simulink model "ultra"  (R2020b)
settings: Solver=FixedStepDiscrete  StartTime=0.0  StopTime=10.0  FixedStep=0.0005  RelTol=1e-3  EnableMultiTasking=on
undefined symbols (not defined in the file): acc_calmax1, acc_calmax2, acc_calmin1, acc_calmin2, akemancanshu, bre, bre_calmax, bre_calmin, ecucoder_acal, I_AN01_5K1, I_AN03_5V, I_AN04_5V, kd, ki, kp, leftmax, O_SW06_HS1A, rightmax, T_add, T_del, tiaoshi, zhiling
libraries: ec5744lib x215, canmsglib x75, simulink x10
(part 2 of 7)

== system ultra/RX/转向——receive编码器 ==
  CANReceive1 : ec5744lib/RapidECU_U4B/04CANCommunication/CANReceive  canmodule=1  canbuffer=55  canmessageid=hex2dec('99')  canmessagetype=Standard(11-bit ID)  datalength=8  sampletime=-1
      settings: SourceProductName=ECUCoder for MPC5744
  MeaModule8 : ec5744lib/RapidECU_U4B/07Calibration/MeaModule  signal=CANOK_99
      settings: SourceProductName=ECUCoder for MPC5744
  Subsystem3 : Subsystem
  Terminator3 : Terminator
  wires:
  CANReceive1/1 -> Subsystem3/Trigger
  CANReceive1/4 -> Subsystem3/3(msg)
  CANReceive1/2 -> MeaModule8/1
  CANReceive1/5 -> Terminator3/1
  MeaModule8/1 -> Subsystem3/1(Enable)
  CANReceive1/3 -> Subsystem3/2(ID)

== system ultra/TOWORKSTATION/toworkstation ==
  Enable : EnablePort
  toworkstation : Subsystem

== system ultra/TOWORKSTATION/转向 ==
  Data Store Read : DataStoreRead  DataStoreName=match_model
  MATLAB Function : MATLAB Function  TreatAsAtomicUnit=on
  Subsystem : Subsystem
  wires:
  Data Store Read/1 -> MATLAB Function/1(u)
  MATLAB Function/1(y) -> Subsystem/Enable

== system ultra/TX控制器/Subsystem ==
  Enable : EnablePort
  CAN Pack1 : canmsglib/CAN Pack  Commented=on  CANdbFile=C:\Users\Liu keliang\Desktop\HRT2023\HRT23赛季刘科良\CANdbc\steere.dbc  MsgList=New_Message_1  MsgName=New_Message_1  MsgIDType=Standard (11-bit identifier)  MsgIdentifier=1911  MsgLength=4  Remote=off  ApplyMinMax=off  BusOutput=off  SignalInfo={'huahaizhuanxiangerror','16','16','LE','signed','Standard','0','1','0','-Inf','Inf';'steere','0','16','LE','signed','Standard','0','1','0','-Inf','Inf'}
      settings: SourceProductBaseCode=ME,XP,VN  DataFormat=CANdb specified signals
  CANPackMessage1 : ec5744lib/RapidECU_U4B/04CANCommunication/CANPackMessage  Commented=on  datalength=4  sampletime=-1
      settings: SourceProductName=ECUCoder for MPC5744
  CANTransmit1 : ec5744lib/RapidECU_U4B/04CANCommunication/CANTransmit  Commented=on  canmodule=2  canbuffer=15  canmessageid=hex2dec('777')  canmessagetype=Standard(11-bit ID)  datalength=4  sampletime=-1
      settings: SourceProductName=ECUCoder for MPC5744
  Data Store Read : DataStoreRead  Commented=on  DataStoreName=huahaisteere
  Data Store Read3 : DataStoreRead  Commented=on  DataStoreName=steere
  Data Type Conversion1 : DataTypeConversion  Commented=on  OutDataTypeStr=uint8
  Terminator1 : Terminator  Commented=on
  wires:
  Data Type Conversion1/1 -> CANTransmit1/1
  CANPackMessage1/1 -> Data Type Conversion1/1
  Data Store Read3/1 -> CAN Pack1/1
  CAN Pack1/1 -> CANPackMessage1/1
  CANTransmit1/1 -> Terminator1/1
  Data Store Read/1 -> CAN Pack1/2

== system ultra/TX控制器/Subsystem1 ==
  angle : Inport
  v : Inport  Port=2
  Data Store Read4 : DataStoreRead  DataStoreName=match_model
  ECCalVar : Constant  InitFcn=ecucoder_acal;  Value=akemancanshu  OutDataTypeStr=Inherit: Inherit via back propagation  SampleTime=-1
  MATLAB Function2 : MATLAB Function  TreatAsAtomicUnit=on
  youqianvvv : Outport
  zuoqianvvv : Outport  Port=2
  youhouvvv : Outport  Port=3
  zuohouvvv : Outport  Port=4
  wires:
  MATLAB Function2/2(zuoqianvvv) -> zuoqianvvv/1
  v/1 -> MATLAB Function2/2(v)
  MATLAB Function2/1(youqianvvv) -> youqianvvv/1
  MATLAB Function2/3(youhouvvv) -> youhouvvv/1
  angle/1 -> MATLAB Function2/1(anglenb)
  MATLAB Function2/4(zuohouvvv) -> zuohouvvv/1
  Data Store Read4/1 -> MATLAB Function2/3(model)
  ECCalVar/1 -> MATLAB Function2/4(k)

== system ultra/TX控制器/扭矩 ==
  Enable : EnablePort
  184左前 : Subsystem
  185右前 : Subsystem
  188右后 : Subsystem
  189左后 : Subsystem
  TEST : Subsystem

== system ultra/TX控制器/速度 ==
  Enable : EnablePort
  184左前 : Subsystem
  185右前 : Subsystem
  188右后 : Subsystem
  189左后 : Subsystem

== system ultra/esc,ABS/Subsystem ==
  Enable : EnablePort
  CAN Pack : canmsglib/CAN Pack  CANdbFile=C:\Users\Liu keliang\Desktop\HRT2023\HRT23赛季刘科良\CANdbc\esc.dbc  MsgList=esc  MsgName=esc  MsgIDType=Standard (11-bit identifier)  MsgIdentifier=1638  MsgLength=8  Remote=off  ApplyMinMax=off  BusOutput=off  SignalInfo={'youhou','0','16','LE','unsigned','Standard','0','1','0','0','65535';'youqian','16','16','LE','unsigned','Standard','0','1','0','0','65535';'zuohou','32','16','LE','unsigned','Standard','0','1','0','0','65535';'zuoqian','48','16','LE','unsigned','Standard','0','1','0','0','65535'}
      settings: SourceProductBaseCode=ME,XP,VN  DataFormat=CANdb specified signals
  CANPackMessage : ec5744lib/RapidECU_U4B/04CANCommunication/CANPackMessage  datalength=8  sampletime=-1
      settings: SourceProductName=ECUCoder for MPC5744
  CANTransmit : ec5744lib/RapidECU_U4B/04CANCommunication/CANTransmit  canmodule=2  canbuffer=12  canmessageid=hex2dec('666')  canmessagetype=Standard(11-bit ID)  datalength=8  sampletime=-1
      settings: SourceProductName=ECUCoder for MPC5744
  Data Store Read : DataStoreRead  DataStoreName=oral_pressure_leftbehind
  Data Store Read1 : DataStoreRead  DataStoreName=oral_pressure_rightbehind
  Data Store Read2 : DataStoreRead  DataStoreName=oral_pressure_rightfront
  Data Store Read3 : DataStoreRead  DataStoreName=oral_pressure_leftfront
  Data Store Read4 : DataStoreRead  DataStoreName=brake_slipzuohou
  Data Store Read5 : DataStoreRead  DataStoreName=brake_slipyouhou
  Data Store Read6 : DataStoreRead  DataStoreName=brake_slipyouqian
  Data Store Read7 : DataStoreRead  DataStoreName=brake_slipzuoqian
  Data Store Read8 : DataStoreRead  DataStoreName=workstation_status
  Data Type Conversion : DataTypeConversion  OutDataTypeStr=uint8
  MATLAB Function : MATLAB Function  TreatAsAtomicUnit=on
  MATLAB Function1 : MATLAB Function  TreatAsAtomicUnit=on
  MATLAB Function2 : MATLAB Function  TreatAsAtomicUnit=on
  MATLAB Function3 : MATLAB Function  TreatAsAtomicUnit=on
  Max{,1..3} (4 alike) : MinMax  Function=max  Inputs=2
  MeaModule : ec5744lib/RapidECU_U4B/07Calibration/MeaModule  signal=esc
      settings: SourceProductName=ECUCoder for MPC5744
  Terminator : Terminator
  wires:
  CAN Pack/1 -> CANPackMessage/1
  CANTransmit/1 -> MeaModule/1
  Data Type Conversion/1 -> CANTransmit/1
  CANPackMessage/1 -> Data Type Conversion/1
  MeaModule/1 -> Terminator/1
  Data Store Read5/1 -> Max/1
  Data Store Read1/1 -> Max/2
  Data Store Read2/1 -> Max1/1
  Data Store Read6/1 -> Max1/2
  Data Store Read/1 -> Max2/1
  Data Store Read4/1 -> Max2/2
  Data Store Read7/1 -> Max3/1
  Data Store Read3/1 -> Max3/2
  Data Store Read8/1 -> MATLAB Function/2(status), MATLAB Function3/2(status), MATLAB Function2/2(status), MATLAB Function1/2(status)
  Max/1 -> MATLAB Function/1(u)
  Max1/1 -> MATLAB Function1/1(u)
  Max2/1 -> MATLAB Function2/1(u)
  Max3/1 -> MATLAB Function3/1(u)
  MATLAB Function/1(y) -> CAN Pack/1
  MATLAB Function1/1(y) -> CAN Pack/2
  MATLAB Function2/1(y) -> CAN Pack/3
  MATLAB Function3/1(y) -> CAN Pack/4

== system ultra/run/analog_input ==
  Add : Sum
  Data Store Read : DataStoreRead  DataStoreName=isdriveless
  Data Store Read{1..3,7} (4 alike) : DataStoreRead  DataStoreName=match_model
  Data Store Read4 : DataStoreRead  DataStoreName=lcu_canok
  Data Store Read5 : DataStoreRead  DataStoreName=lcu_canok
  Data Store Read6 : DataStoreRead  DataStoreName=workstation_status
  Data Store Read8 : DataStoreRead  DataStoreName=V_workstation
  Data Store Read9 : DataStoreRead  DataStoreName=V_Kalman
  Data Store Write : DataStoreWrite  DataStoreName=M
  MATLAB Function : MATLAB Function  TreatAsAtomicUnit=on
  MATLAB Function1 : MATLAB Function  TreatAsAtomicUnit=on
  MATLAB Function2 : MATLAB Function  TreatAsAtomicUnit=on
  MATLAB Function3 : MATLAB Function  TreatAsAtomicUnit=on
  MATLAB Function4 : MATLAB Function  TreatAsAtomicUnit=on
  MATLAB Function5 : MATLAB Function  TreatAsAtomicUnit=on
  Saturation : Saturate  UpperLimit=50  LowerLimit=0
  Switch : Switch  Criteria=u2 > Threshold
  无人意图转译 : Subsystem
  有人 : Subsystem
  bre : Outport
  acc : Outport  Port=2
  wires:
  Data Store Read1/1 -> MATLAB Function/1(u)
  MATLAB Function/1(y) -> MATLAB Function1/1(u)
  Switch/1 -> MATLAB Function1/2(a)
  有人/1(TP) -> Switch/3
  有人/2(bre) -> bre/1
  Data Store Read2/1 -> MATLAB Function2/1(u)
  MATLAB Function2/1(y) -> 有人/Enable
  Data Store Read3/1 -> MATLAB Function3/1(u)
  无人意图转译/1(Out1) -> Switch/1
  MATLAB Function3/1(y) -> 无人意图转译/Enable
  Data Store Read4/1 -> MATLAB Function3/2(canok)
  Data Store Read5/1 -> MATLAB Function2/2(canok)
  Data Store Read6/1 -> MATLAB Function4/1(u)
  MATLAB Function1/1(y) -> MATLAB Function4/2(a)
  MATLAB Function4/1(y) -> MATLAB Function5/1(u)
  Data Store Read7/1 -> MATLAB Function5/2(model)
  MATLAB Function5/2(y6) -> Saturation/1
  Saturation/1 -> Add/2
  MATLAB Function5/1(y) -> Add/1
  Add/1 -> Data Store Write/1, acc/1
  Data Store Read/1 -> Switch/2
  Data Store Read8/1 -> MATLAB Function3/3(workstation)
  Data Store Read9/1 -> MATLAB Function3/4(v)

== system ultra/run/ctrl ==
  note: 控制策略所在地
  基准扭矩 : Inport
  Subsystem1 : Subsystem
  wires:
  基准扭矩/1 -> Subsystem1/1(扭矩)

== system ultra/无人TX/转向换算 ==
  Enable : EnablePort
  Data Store Read : DataStoreRead  DataStoreName=zhuanxiangbaocuo
  Data Store Read1 : DataStoreRead  DataStoreName=zhuanxiangbaocuo
  MATLAB Function : MATLAB Function  TreatAsAtomicUnit=on
  MATLAB Function1 : MATLAB Function  TreatAsAtomicUnit=on
  Subsystem : Subsystem
  Subsystem1 : Subsystem
  wires:
  MATLAB Function/1(biaozhi1) -> Subsystem/Enable
  MATLAB Function1/3(biaozhi2) -> Subsystem1/Enable
  MATLAB Function1/2(y2) -> Subsystem1/2(y2)
  MATLAB Function1/1(y1) -> Subsystem1/1(y1)
  Data Store Read/1 -> MATLAB Function1/1(baocuo)
  Data Store Read1/1 -> MATLAB Function/1(baocuo)

== system ultra/转向自动标定/转向自动标定 ==
  Enable : EnablePort
  MATLAB Function : MATLAB Function  TreatAsAtomicUnit=on
  MATLAB Function1 : MATLAB Function  TreatAsAtomicUnit=on
  Subsystem : Subsystem
  Subsystem1 : Subsystem
  wires:
  MATLAB Function/1(biaozhi1) -> Subsystem/Enable
  MATLAB Function1/3(biaozhi2) -> Subsystem1/Enable
  MATLAB Function1/2(y2) -> Subsystem1/2(y2)
  MATLAB Function1/1(y1) -> Subsystem1/1(y1)

== system ultra/RX/283 285左前/Subsystem1 ==
  Enable : Inport
  ID : Inport  Port=2
  msg : Inport  Port=3
  function : TriggerPort  TriggerType=function-call  VariantControl=Variant
  Subsystem : Subsystem
  wires:
  ID/1 -> Subsystem/1(ID)
  msg/1 -> Subsystem/2(msg)
  Enable/1 -> Subsystem/Enable

== system ultra/RX/283 285左前/Subsystem2 ==
  Enable : Inport
  ID : Inport  Port=2
  msg : Inport  Port=3
  function : TriggerPort  TriggerType=function-call  VariantControl=Variant
  Subsystem : Subsystem
  wires:
  ID/1 -> Subsystem/1(ID)
  msg/1 -> Subsystem/2(msg)
  Enable/1 -> Subsystem/Enable

== system ultra/RX/284 286右前/Subsystem1 ==
  Enable : Inport
  ID : Inport  Port=2
  msg : Inport  Port=3
  function : TriggerPort  TriggerType=function-call  VariantControl=Variant
  Subsystem : Subsystem
  wires:
  ID/1 -> Subsystem/1(ID)
  msg/1 -> Subsystem/2(msg)
  Enable/1 -> Subsystem/Enable

== system ultra/RX/284 286右前/Subsystem2 ==
  Enable : Inport
  ID : Inport  Port=2
  msg : Inport  Port=3
  function : TriggerPort  TriggerType=function-call  VariantControl=Variant
  Subsystem : Subsystem
  wires:
  ID/1 -> Subsystem/1(ID)
  msg/1 -> Subsystem/2(msg)
  Enable/1 -> Subsystem/Enable

== system ultra/RX/287 289右后/Subsystem1 ==
  Enable : Inport
  ID : Inport  Port=2
  msg : Inport  Port=3
  function : TriggerPort  TriggerType=function-call  VariantControl=Variant
  Subsystem : Subsystem
  wires:
  ID/1 -> Subsystem/1(ID)
  msg/1 -> Subsystem/2(msg)
  Enable/1 -> Subsystem/Enable

== system ultra/RX/287 289右后/Subsystem2 ==
  Enable : Inport
  ID : Inport  Port=2
  msg : Inport  Port=3
  function : TriggerPort  TriggerType=function-call  VariantControl=Variant
  Subsystem : Subsystem
  wires:
  ID/1 -> Subsystem/1(ID)
  msg/1 -> Subsystem/2(msg)
  Enable/1 -> Subsystem/Enable

== system ultra/RX/287 289右后/Subsystem3 ==
  Enable : Inport
  ID : Inport  Port=2
  msg : Inport  Port=3
  function : TriggerPort  TriggerType=function-call  VariantControl=Variant
  Subsystem : Subsystem
  wires:
  ID/1 -> Subsystem/1(ID)
  msg/1 -> Subsystem/2(msg)
  Enable/1 -> Subsystem/Enable

== system ultra/RX/288 290左后/Subsystem1 ==
  Enable : Inport
  ID : Inport  Port=2
  msg : Inport  Port=3
  function : TriggerPort  TriggerType=function-call  VariantControl=Variant
  Subsystem : Subsystem
  wires:
  ID/1 -> Subsystem/1(ID)
  msg/1 -> Subsystem/2(msg)
  Enable/1 -> Subsystem/Enable

== system ultra/RX/288 290左后/Subsystem2 ==
  Enable : Inport
  ID : Inport  Port=2
  msg : Inport  Port=3
  function : TriggerPort  TriggerType=function-call  VariantControl=Variant
  Subsystem : Subsystem
  wires:
  ID/1 -> Subsystem/1(ID)
  msg/1 -> Subsystem/2(msg)
  Enable/1 -> Subsystem/Enable

== system ultra/RX/ebs/Subsystem3 ==
  Enable : Inport
  ID : Inport  Port=2
  msg : Inport  Port=3
  function : TriggerPort  TriggerType=function-call  VariantControl=Variant
  Subsystem : Subsystem
  wires:
  ID/1 -> Subsystem/1(ID)
  msg/1 -> Subsystem/2(msg)
  Enable/1 -> Subsystem/Enable

== system ultra/RX/lcu——receive/Subsystem1 ==
  Enable : Inport
  ID : Inport  Port=2
  msg : Inport  Port=3
  function : TriggerPort  TriggerType=function-call  VariantControl=Variant
  Subsystem : Subsystem
  Out1 : Outport
  m : Outport  Port=2
  wires:
  ID/1 -> Subsystem/1(ID)
  msg/1 -> Subsystem/2(msg)
  Subsystem/1(Out1) -> Out1/1
  Enable/1 -> Subsystem/Enable
  Subsystem/2(CAN_msg_enable) -> m/1

== system ultra/RX/工作站/Subsystem1 ==
  Enable : Inport
  ID : Inport  Port=2
  msg : Inport  Port=3
  function : TriggerPort  TriggerType=function-call  VariantControl=Variant
  Subsystem1 : Subsystem
  wires:
  Enable/1 -> Subsystem1/Enable
  ID/1 -> Subsystem1/1(ID)
  msg/1 -> Subsystem1/2(msg)

== system ultra/RX/工作站/Subsystem3 ==
  Enable : Inport
  ID : Inport  Port=2
  msg : Inport  Port=3
  function : TriggerPort  TriggerType=function-call  VariantControl=Variant
  Subsystem : Subsystem
  wires:
  ID/1 -> Subsystem/1(ID)
  msg/1 -> Subsystem/2(msg)
  Enable/1 -> Subsystem/Enable

== system ultra/RX/惯导/Subsystem1 ==
  Enable : Inport
  ID : Inport  Port=2
  msg : Inport  Port=3
  function : TriggerPort  TriggerType=function-call  VariantControl=Variant
  Subsystem : Subsystem
  wires:
  ID/1 -> Subsystem/1(ID)
  msg/1 -> Subsystem/2(msg)
  Enable/1 -> Subsystem/Enable

== system ultra/RX/惯导/Subsystem2 ==
  Enable : Inport
  ID : Inport  Port=2
  msg : Inport  Port=3
  function : TriggerPort  TriggerType=function-call  VariantControl=Variant
  Subsystem : Subsystem
  wires:
  ID/1 -> Subsystem/1(ID)
  msg/1 -> Subsystem/2(msg)
  Enable/1 -> Subsystem/Enable

== system ultra/RX/惯导/Subsystem3 ==
  Enable : Inport
  ID : Inport  Port=2
  msg : Inport  Port=3
  function : TriggerPort  TriggerType=function-call  VariantControl=Variant
  Subsystem : Subsystem
  wires:
  ID/1 -> Subsystem/1(ID)
  msg/1 -> Subsystem/2(msg)
  Enable/1 -> Subsystem/Enable

== system ultra/RX/转向——receive1/Subsystem1 ==
  Enable : Inport
  ID : Inport  Port=2
  msg : Inport  Port=3
  function : TriggerPort  TriggerType=function-call  VariantControl=Variant
  Subsystem : Subsystem
  wires:
  ID/1 -> Subsystem/1(ID)
  msg/1 -> Subsystem/2(msg)
  Enable/1 -> Subsystem/Enable

== system ultra/RX/转向——receive1/Subsystem3 ==
  Enable : Inport
  ID : Inport  Port=2
  msg : Inport  Port=3
  function : TriggerPort  TriggerType=function-call  VariantControl=Variant
  Subsystem : Subsystem
  wires:
  ID/1 -> Subsystem/1(ID)
  msg/1 -> Subsystem/2(msg)
  Enable/1 -> Subsystem/Enable

== system ultra/RX/转向——receive编码器/Subsystem3 ==
  Enable : Inport
  ID : Inport  Port=2
  msg : Inport  Port=3
  function : TriggerPort  TriggerType=function-call  VariantControl=Variant
  Subsystem : Subsystem
  wires:
  ID/1 -> Subsystem/1(ID)
  msg/1 -> Subsystem/2(msg)
  Enable/1 -> Subsystem/Enable

== system ultra/TOWORKSTATION/toworkstation/toworkstation ==
  CAN Pack : canmsglib/CAN Pack  CANdbFile=C:\Users\Liu keliang\Desktop\HRT2023\HRT23赛季刘科良\CANdbc\toworkstation.dbc  MsgList=toworkstation  MsgName=toworkstation  MsgIDType=Standard (11-bit identifier)  MsgIdentifier=562  MsgLength=8  Remote=off  ApplyMinMax=off  BusOutput=off  SignalInfo={'youhou','0','16','LE','signed','Standard','0','1','0','-Inf','Inf';'youqian','16','16','LE','signed','Standard','0','1','0','-Inf','Inf';'zuohou','32','16','LE','signed','Standard','0','1','0','-Inf','Inf';'zuoqian','48','16','LE','signed','Standard','0','1','0','-Inf','Inf'}
      settings: SourceProductBaseCode=ME,XP,VN  DataFormat=CANdb specified signals
  CAN Pack1 : canmsglib/CAN Pack  CANdbFile=C:\Users\Liu keliang\Desktop\HRT2023\HRT23赛季刘科良\CANdbc\ecuangle.dbc  MsgList=New_Message_1  MsgName=New_Message_1  MsgIDType=Standard (11-bit identifier)  MsgIdentifier=563  MsgLength=2  Remote=off  ApplyMinMax=off  BusOutput=off  SignalInfo={'New_Signal_1','0','16','LE','signed','Standard','0','1','0','-1080','1080';'angelerror','16','8','LE','signed','Standard','0','1','0','-Inf','Inf'}
      settings: SourceProductBaseCode=ME,XP,VN  DataFormat=CANdb specified signals
  CANPackMessage : ec5744lib/RapidECU_U4B/04CANCommunication/CANPackMessage  datalength=8  sampletime=-1
      settings: SourceProductName=ECUCoder for MPC5744
  CANPackMessage1 : ec5744lib/RapidECU_U4B/04CANCommunication/CANPackMessage  datalength=2  sampletime=-1
      settings: SourceProductName=ECUCoder for MPC5744
  CANTransmit : ec5744lib/RapidECU_U4B/04CANCommunication/CANTransmit  canmodule=2  canbuffer=59  canmessageid=hex2dec('232')  canmessagetype=Standard(11-bit ID)  datalength=8  sampletime=-1
      settings: SourceProductName=ECUCoder for MPC5744
  CANTransmit1 : ec5744lib/RapidECU_U4B/04CANCommunication/CANTransmit  canmodule=2  canbuffer=63  canmessageid=hex2dec('233')  canmessagetype=Standard(11-bit ID)  datalength=2  sampletime=-1
      settings: SourceProductName=ECUCoder for MPC5744
  Data Store Read : DataStoreRead  DataStoreName=dianji_velcoity_zuoqian1
  Data Store Read1 : DataStoreRead  DataStoreName=dianji_velcoity_youhou1
  Data Store Read2 : DataStoreRead  DataStoreName=dianji_velcoity_youqian1
  Data Store Read3 : DataStoreRead  DataStoreName=dianji_velcoity_zuohou1
  Data Store Read4 : DataStoreRead  DataStoreName=zhuanjiaoweigeniubi
  Data Store Read5 : DataStoreRead  DataStoreName=steere
  Data Type Conversion : DataTypeConversion  OutDataTypeStr=uint8
  Data Type Conversion1 : DataTypeConversion  OutDataTypeStr=uint8
  MeaModule : ec5744lib/RapidECU_U4B/07Calibration/MeaModule  signal=T232
      settings: SourceProductName=ECUCoder for MPC5744
  MeaModule1 : ec5744lib/RapidECU_U4B/07Calibration/MeaModule  signal=T233
      settings: SourceProductName=ECUCoder for MPC5744
  Terminator : Terminator
  Terminator1 : Terminator
  wires:
  CANPackMessage/1 -> Data Type Conversion/1
  CAN Pack/1 -> CANPackMessage/1
  CANTransmit/1 -> MeaModule/1
  MeaModule/1 -> Terminator/1
  Data Type Conversion/1 -> CANTransmit/1
  Data Store Read/1 -> CAN Pack/4
  Data Store Read1/1 -> CAN Pack/1
  Data Store Read2/1 -> CAN Pack/2
  Data Store Read3/1 -> CAN Pack/3
  CANTransmit1/1 -> MeaModule1/1
  MeaModule1/1 -> Terminator1/1
  CANPackMessage1/1 -> Data Type Conversion1/1
  CAN Pack1/1 -> CANPackMessage1/1
  Data Type Conversion1/1 -> CANTransmit1/1
  Data Store Read4/1 -> CAN Pack1/1
  Data Store Read5/1 -> CAN Pack1/2

== system ultra/TOWORKSTATION/转向/Subsystem ==
  Enable : EnablePort
  MATLAB Function : MATLAB Function  TreatAsAtomicUnit=on
  MATLAB Function1 : MATLAB Function  TreatAsAtomicUnit=on
  Subsystem : Subsystem
  Subsystem1 : Subsystem
  wires:
  MATLAB Function/1(biaozhi1) -> Subsystem/Enable
  MATLAB Function1/2(y2) -> Subsystem1/2(y2)
  MATLAB Function1/1(y1) -> Subsystem1/1(y1)
  MATLAB Function1/3(biaozhi2) -> Subsystem1/Enable

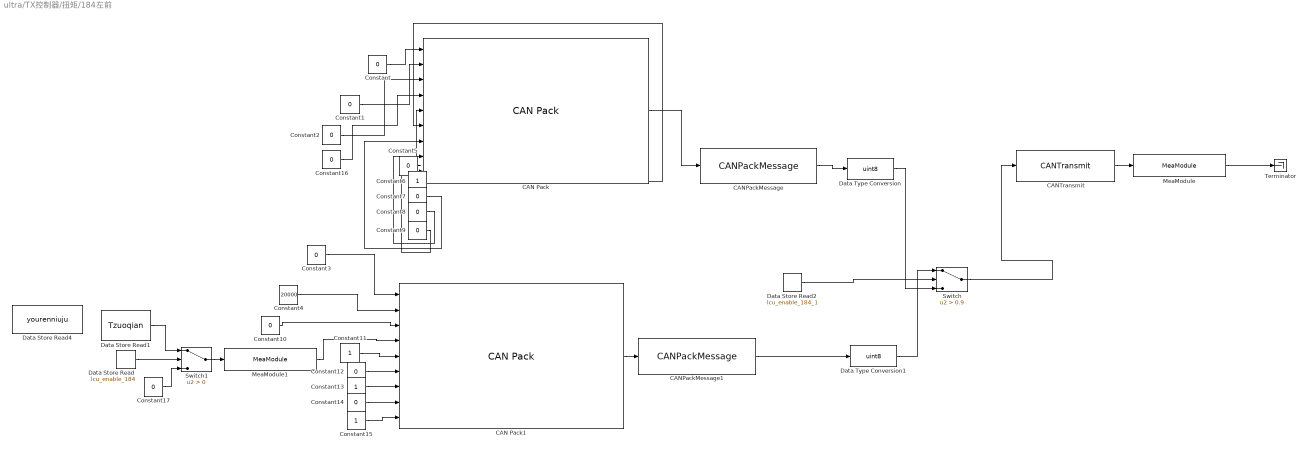
== system ultra/TX控制器/扭矩/184左前 ==
  CAN Pack : canmsglib/CAN Pack  CANdbFile=D:\desktop\CANdbc\enable.dbc  MsgList=(none)  MsgName=first_enable  MsgIDType=Standard (11-bit identifier)  MsgIdentifier=388  MsgLength=8  Remote=off  ApplyMinMax=off  BusOutput=off  SignalInfo={'AMK_Reserve','12','4','LE','signed','Standard','0','1','0','0','15';'AMK_TargetVelocity','16','16','LE','signed','Standard','0','1','0','0','65535';'AMK_TorqueLimitNegativ','48','16','LE','signed','Standard','0','1','0','0','65535';'AMK_TorqueLimitPositiv','32','16','LE','signed','Standard','0','1','0','0','65535';'AMK_bEnable','10','1','LE','unsigned','Standard','0','1','0','0','1';'AMK_bErrorReset','11','1','LE','unsigned','Standard','0','1','0','0','1';'AMK_bInverterOn','8','1','LE','unsigned','Standard','0','1','0','0','1';'AMK_bReserve','0','8','LE','unsigned','Standard','0','1','0','0','255';'CAN_bdcon','9','1','LE','unsigned','Standard','0','1','0','0','1'}
      settings: SourceProductBaseCode=ME,XP,VN  DataFormat=CANdb specified signals
  CAN Pack1 : canmsglib/CAN Pack  CANdbFile=D:\desktop\CANdbc\enable.dbc  MsgList=(none)  MsgName=first_enable  MsgIDType=Standard (11-bit identifier)  MsgIdentifier=388  MsgLength=8  Remote=off  ApplyMinMax=off  BusOutput=off  SignalInfo={'AMK_Reserve','12','4','LE','signed','Standard','0','1','0','0','15';'AMK_TargetVelocity','16','16','LE','signed','Standard','0','1','0','0','65535';'AMK_TorqueLimitNegativ','48','16','LE','signed','Standard','0','1','0','0','65535';'AMK_TorqueLimitPositiv','32','16','LE','signed','Standard','0','1','0','0','65535';'AMK_bEnable','10','1','LE','unsigned','Standard','0','1','0','0','1';'AMK_bErrorReset','11','1','LE','unsigned','Standard','0','1','0','0','1';'AMK_bInverterOn','8','1','LE','unsigned','Standard','0','1','0','0','1';'AMK_bReserve','0','8','LE','unsigned','Standard','0','1','0','0','255';'CAN_bdcon','9','1','LE','unsigned','Standard','0','1','0','0','1'}
      settings: SourceProductBaseCode=ME,XP,VN  DataFormat=CANdb specified signals
  CANPackMessage : ec5744lib/RapidECU_U4B/04CANCommunication/CANPackMessage  datalength=8  sampletime=-1
      settings: SourceProductName=ECUCoder for MPC5744
  CANPackMessage1 : ec5744lib/RapidECU_U4B/04CANCommunication/CANPackMessage  datalength=8  sampletime=-1
      settings: SourceProductName=ECUCoder for MPC5744
  CANTransmit : ec5744lib/RapidECU_U4B/04CANCommunication/CANTransmit  canmodule=0  canbuffer=8  canmessageid=hex2dec('184')  canmessagetype=Standard(11-bit ID)  datalength=8  sampletime=-1
      settings: SourceProductName=ECUCoder for MPC5744
  Constant{,1..3,5,7..10,12,14,16..17} (13 alike) : Constant  Value=0  SampleTime=-1
  Constant{6,11,13,15} (4 alike) : Constant  SampleTime=-1
  Constant4 : Constant  Value=20000  SampleTime=-1
  Data Store Read : DataStoreRead  DataStoreName=lcu_enable_184
  Data Store Read1 : DataStoreRead  DataStoreName=Tzuoqian
  Data Store Read2 : DataStoreRead  DataStoreName=lcu_enable_184_1
  Data Store Read4 : DataStoreRead  DataStoreName=yourenniuju
  Data Type Conversion : DataTypeConversion  OutDataTypeStr=uint8
  Data Type Conversion1 : DataTypeConversion  OutDataTypeStr=uint8
  MeaModule : ec5744lib/RapidECU_U4B/07Calibration/MeaModule  signal=T184
      settings: SourceProductName=ECUCoder for MPC5744
  MeaModule1 : ec5744lib/RapidECU_U4B/07Calibration/MeaModule  signal=Tfirst
      settings: SourceProductName=ECUCoder for MPC5744
  Switch : Switch  Criteria=u2 > Threshold  Threshold=0.9
  Switch1 : Switch  Criteria=u2 > Threshold
  Terminator : Terminator
  wires:
  Constant8/1 -> CAN Pack/8
  Constant5/1 -> CAN Pack/5
  Constant/1 -> CAN Pack/1
  Constant9/1 -> CAN Pack/9
  CAN Pack/1 -> CANPackMessage/1
  Constant7/1 -> CAN Pack/7
  Constant1/1 -> CAN Pack/2
  Constant16/1 -> CAN Pack/4
  Constant2/1 -> CAN Pack/3
  Constant6/1 -> CAN Pack/6
  CANTransmit/1 -> MeaModule/1
  MeaModule/1 -> Terminator/1
  Constant14/1 -> CAN Pack1/8
  Constant3/1 -> CAN Pack1/1
  Constant13/1 -> CAN Pack1/7
  CAN Pack1/1 -> CANPackMessage1/1
  Constant12/1 -> CAN Pack1/6
  CANPackMessage1/1 -> Data Type Conversion1/1
  Constant4/1 -> CAN Pack1/2
  Constant15/1 -> CAN Pack1/9
  Constant11/1 -> CAN Pack1/5
  Data Type Conversion1/1 -> Switch/1
  Constant10/1 -> CAN Pack1/3
  Switch/1 -> CANTransmit/1
  CANPackMessage/1 -> Data Type Conversion/1
  Data Type Conversion/1 -> Switch/3
  MeaModule1/1 -> CAN Pack1/4
  Switch1/1 -> MeaModule1/1
  Data Store Read/1 -> Switch1/2
  Constant17/1 -> Switch1/3
  Data Store Read2/1 -> Switch/2
  Data Store Read1/1 -> Switch1/1

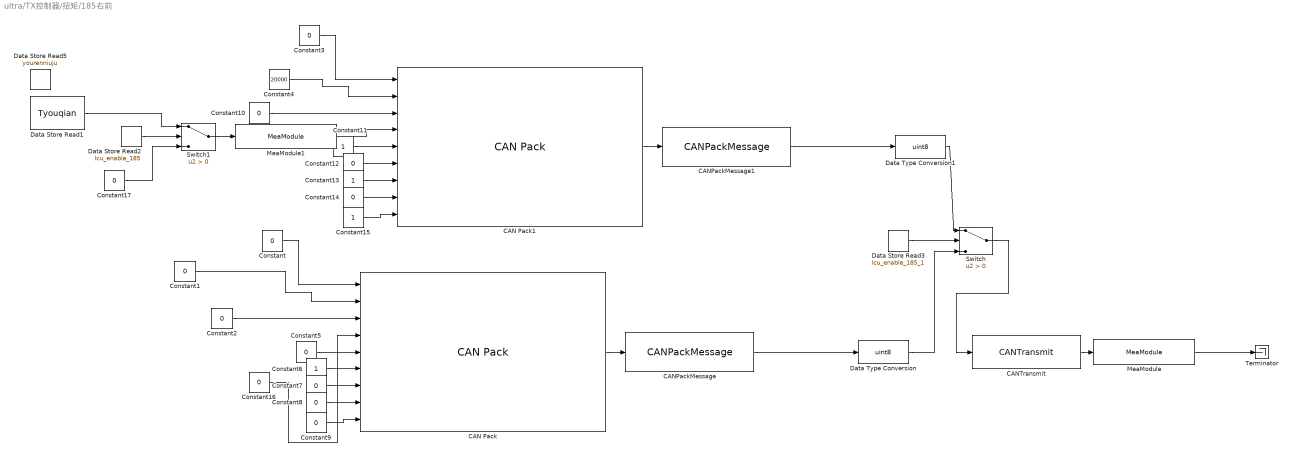
== system ultra/TX控制器/扭矩/185右前 ==
  CAN Pack : canmsglib/CAN Pack  CANdbFile=D:\desktop\CANdbc\enable - youqian.dbc  MsgList=(none)  MsgName=first_enable  MsgIDType=Standard (11-bit identifier)  MsgIdentifier=389  MsgLength=8  Remote=off  ApplyMinMax=off  BusOutput=off  SignalInfo={'AMK_Reserve','12','4','LE','signed','Standard','0','1','0','0','15';'AMK_TargetVelocity','16','16','LE','signed','Standard','0','1','0','0','65535';'AMK_TorqueLimitNegativ','48','16','LE','signed','Standard','0','1','0','0','65535';'AMK_TorqueLimitPositiv','32','16','LE','signed','Standard','0','1','0','0','65535';'AMK_bEnable','10','1','LE','unsigned','Standard','0','1','0','0','1';'AMK_bErrorReset','11','1','LE','unsigned','Standard','0','1','0','0','1';'AMK_bInverterOn','8','1','LE','unsigned','Standard','0','1','0','0','1';'AMK_bReserve','0','8','LE','unsigned','Standard','0','1','0','0','255';'CAN_bdcon','9','1','LE','unsigned','Standard','0','1','0','0','1'}
      settings: SourceProductBaseCode=ME,XP,VN  DataFormat=CANdb specified signals
  CAN Pack1 : canmsglib/CAN Pack  CANdbFile=D:\desktop\CANdbc\enable - youqian.dbc  MsgList=(none)  MsgName=first_enable  MsgIDType=Standard (11-bit identifier)  MsgIdentifier=389  MsgLength=8  Remote=off  ApplyMinMax=off  BusOutput=off  SignalInfo={'AMK_Reserve','12','4','LE','signed','Standard','0','1','0','0','15';'AMK_TargetVelocity','16','16','LE','signed','Standard','0','1','0','0','65535';'AMK_TorqueLimitNegativ','48','16','LE','signed','Standard','0','1','0','0','65535';'AMK_TorqueLimitPositiv','32','16','LE','signed','Standard','0','1','0','0','65535';'AMK_bEnable','10','1','LE','unsigned','Standard','0','1','0','0','1';'AMK_bErrorReset','11','1','LE','unsigned','Standard','0','1','0','0','1';'AMK_bInverterOn','8','1','LE','unsigned','Standard','0','1','0','0','1';'AMK_bReserve','0','8','LE','unsigned','Standard','0','1','0','0','255';'CAN_bdcon','9','1','LE','unsigned','Standard','0','1','0','0','1'}
      settings: SourceProductBaseCode=ME,XP,VN  DataFormat=CANdb specified signals
  CANPackMessage : ec5744lib/RapidECU_U4B/04CANCommunication/CANPackMessage  datalength=8  sampletime=-1
      settings: SourceProductName=ECUCoder for MPC5744
  CANPackMessage1 : ec5744lib/RapidECU_U4B/04CANCommunication/CANPackMessage  datalength=8  sampletime=-1
      settings: SourceProductName=ECUCoder for MPC5744
  CANTransmit : ec5744lib/RapidECU_U4B/04CANCommunication/CANTransmit  canmodule=0  canbuffer=11  canmessageid=hex2dec('185')  canmessagetype=Standard(11-bit ID)  datalength=8  sampletime=-1
      settings: SourceProductName=ECUCoder for MPC5744
  Constant{,1..3,5,7..10,12,14,16..17} (13 alike) : Constant  Value=0  SampleTime=-1
  Constant{6,11,13,15} (4 alike) : Constant  SampleTime=-1
  Constant4 : Constant  Value=20000  SampleTime=-1
  Data Store Read1 : DataStoreRead  DataStoreName=Tyouqian
  Data Store Read2 : DataStoreRead  DataStoreName=lcu_enable_185
  Data Store Read3 : DataStoreRead  DataStoreName=lcu_enable_185_1
  Data Store Read5 : DataStoreRead  DataStoreName=yourenniuju
  Data Type Conversion : DataTypeConversion  OutDataTypeStr=uint8
  Data Type Conversion1 : DataTypeConversion  OutDataTypeStr=uint8
  MeaModule : ec5744lib/RapidECU_U4B/07Calibration/MeaModule  signal=T185
      settings: SourceProductName=ECUCoder for MPC5744
  MeaModule1 : ec5744lib/RapidECU_U4B/07Calibration/MeaModule  signal=Tforth
      settings: SourceProductName=ECUCoder for MPC5744
  Switch : Switch  Criteria=u2 > Threshold
  Switch1 : Switch  Criteria=u2 > Threshold
  Terminator : Terminator
  wires:
  Constant8/1 -> CAN Pack/8
  Constant5/1 -> CAN Pack/5
  Constant/1 -> CAN Pack/1
  CANPackMessage/1 -> Data Type Conversion/1
  Constant9/1 -> CAN Pack/9
  CAN Pack/1 -> CANPackMessage/1
  Constant7/1 -> CAN Pack/7
  Constant1/1 -> CAN Pack/2
  Constant16/1 -> CAN Pack/4
  Constant2/1 -> CAN Pack/3
  Constant6/1 -> CAN Pack/6
  CANTransmit/1 -> MeaModule/1
  MeaModule/1 -> Terminator/1
  CANPackMessage1/1 -> Data Type Conversion1/1
  Constant3/1 -> CAN Pack1/1
  Constant11/1 -> CAN Pack1/5
  Constant12/1 -> CAN Pack1/6
  Constant13/1 -> CAN Pack1/7
  CAN Pack1/1 -> CANPackMessage1/1
  Constant10/1 -> CAN Pack1/3
  Constant14/1 -> CAN Pack1/8
  Constant4/1 -> CAN Pack1/2
  Constant15/1 -> CAN Pack1/9
  Data Type Conversion1/1 -> Switch/1
  Data Type Conversion/1 -> Switch/3
  Switch/1 -> CANTransmit/1
  Data Store Read3/1 -> Switch/2
  MeaModule1/1 -> CAN Pack1/4
  Switch1/1 -> MeaModule1/1
  Constant17/1 -> Switch1/3
  Data Store Read2/1 -> Switch1/2
  Data Store Read1/1 -> Switch1/1

== system ultra/TX控制器/扭矩/188右后 ==
  CAN Pack : canmsglib/CAN Pack  CANdbFile=D:\desktop\CANdbc\enable - zuohou - 副本.dbc  MsgList=(none)  MsgName=first_enable  MsgIDType=Standard (11-bit identifier)  MsgIdentifier=392  MsgLength=8  Remote=off  ApplyMinMax=off  BusOutput=off  SignalInfo={'AMK_Reserve','12','4','LE','signed','Standard','0','1','0','0','15';'AMK_TargetVelocity','16','16','LE','signed','Standard','0','1','0','0','65535';'AMK_TorqueLimitNegativ','48','16','LE','signed','Standard','0','1','0','0','65535';'AMK_TorqueLimitPositiv','32','16','LE','signed','Standard','0','1','0','0','65535';'AMK_bEnable','10','1','LE','unsigned','Standard','0','1','0','0','1';'AMK_bErrorReset','11','1','LE','unsigned','Standard','0','1','0','0','1';'AMK_bInverterOn','8','1','LE','unsigned','Standard','0','1','0','0','1';'AMK_bReserve','0','8','LE','unsigned','Standard','0','1','0','0','255';'CAN_bdcon','9','1','LE','unsigned','Standard','0','1','0','0','1'}
      settings: SourceProductBaseCode=ME,XP,VN  DataFormat=CANdb specified signals
  CAN Pack1 : canmsglib/CAN Pack  CANdbFile=D:\desktop\CANdbc\enable - zuohou - 副本.dbc  MsgList=(none)  MsgName=first_enable  MsgIDType=Standard (11-bit identifier)  MsgIdentifier=392  MsgLength=8  Remote=off  ApplyMinMax=off  BusOutput=off  SignalInfo={'AMK_Reserve','12','4','LE','signed','Standard','0','1','0','0','15';'AMK_TargetVelocity','16','16','LE','signed','Standard','0','1','0','0','65535';'AMK_TorqueLimitNegativ','48','16','LE','signed','Standard','0','1','0','0','65535';'AMK_TorqueLimitPositiv','32','16','LE','signed','Standard','0','1','0','0','65535';'AMK_bEnable','10','1','LE','unsigned','Standard','0','1','0','0','1';'AMK_bErrorReset','11','1','LE','unsigned','Standard','0','1','0','0','1';'AMK_bInverterOn','8','1','LE','unsigned','Standard','0','1','0','0','1';'AMK_bReserve','0','8','LE','unsigned','Standard','0','1','0','0','255';'CAN_bdcon','9','1','LE','unsigned','Standard','0','1','0','0','1'}
      settings: SourceProductBaseCode=ME,XP,VN  DataFormat=CANdb specified signals
  CANPackMessage : ec5744lib/RapidECU_U4B/04CANCommunication/CANPackMessage  datalength=8  sampletime=-1
      settings: SourceProductName=ECUCoder for MPC5744
  CANPackMessage1 : ec5744lib/RapidECU_U4B/04CANCommunication/CANPackMessage  datalength=8  sampletime=-1
      settings: SourceProductName=ECUCoder for MPC5744
  CANTransmit : ec5744lib/RapidECU_U4B/04CANCommunication/CANTransmit  canmodule=0  canbuffer=9  canmessageid=hex2dec('188')  canmessagetype=Standard(11-bit ID)  datalength=8  sampletime=-1
      settings: SourceProductName=ECUCoder for MPC5744
  Constant{,1..3,5,7..10,12,14,17} (12 alike) : Constant  Value=0  SampleTime=-1
  Constant{6,11,13,15} (4 alike) : Constant  SampleTime=-1
  Constant16 : Constant  Value=0
  Constant4 : Constant  Value=20000  SampleTime=-1
  Data Store Read1 : DataStoreRead  DataStoreName=lcu_enable_188
  Data Store Read2 : DataStoreRead  DataStoreName=Tyouhou
  Data Store Read3 : DataStoreRead  DataStoreName=lcu_enable_188_1
  Data Store Read5 : DataStoreRead  DataStoreName=yourenniuju
  Data Type Conversion : DataTypeConversion  OutDataTypeStr=uint8
  Data Type Conversion1 : DataTypeConversion  OutDataTypeStr=uint8
  MeaModule : ec5744lib/RapidECU_U4B/07Calibration/MeaModule  signal=T188
      settings: SourceProductName=ECUCoder for MPC5744
  MeaModule1 : ec5744lib/RapidECU_U4B/07Calibration/MeaModule  signal=Tsecond
      settings: SourceProductName=ECUCoder for MPC5744
  Switch : Switch  Criteria=u2 > Threshold  Threshold=0.9
  Switch1 : Switch  Criteria=u2 > Threshold
  Terminator : Terminator
  wires:
  Constant8/1 -> CAN Pack/8
  Constant5/1 -> CAN Pack/5
  Constant/1 -> CAN Pack/1
  CANPackMessage/1 -> Data Type Conversion/1
  Constant9/1 -> CAN Pack/9
  CAN Pack/1 -> CANPackMessage/1
  Constant7/1 -> CAN Pack/7
  Constant1/1 -> CAN Pack/2
  Constant16/1 -> CAN Pack/4
  Constant2/1 -> CAN Pack/3
  Constant6/1 -> CAN Pack/6
  CANTransmit/1 -> MeaModule/1
  MeaModule/1 -> Terminator/1
  Data Type Conversion1/1 -> Switch/1
  Constant12/1 -> CAN Pack1/6
  Constant10/1 -> CAN Pack1/3
  Constant4/1 -> CAN Pack1/2
  CANPackMessage1/1 -> Data Type Conversion1/1
  Constant14/1 -> CAN Pack1/8
  Constant3/1 -> CAN Pack1/1
  Constant11/1 -> CAN Pack1/5
  CAN Pack1/1 -> CANPackMessage1/1
  Constant15/1 -> CAN Pack1/9
  Constant13/1 -> CAN Pack1/7
  Data Store Read3/1 -> Switch/2
  Data Type Conversion/1 -> Switch/3
  Switch/1 -> CANTransmit/1
  MeaModule1/1 -> CAN Pack1/4
  Constant17/1 -> Switch1/3
  Data Store Read1/1 -> Switch1/2
  Switch1/1 -> MeaModule1/1
  Data Store Read2/1 -> Switch1/1

== system ultra/TX控制器/扭矩/189左后 ==
  CAN Pack : canmsglib/CAN Pack  CANdbFile=D:\desktop\CANdbc\enable - youhou -.dbc  MsgList=(none)  MsgName=first_enable  MsgIDType=Standard (11-bit identifier)  MsgIdentifier=393  MsgLength=8  Remote=off  ApplyMinMax=off  BusOutput=off  SignalInfo={'AMK_Reserve','12','4','LE','signed','Standard','0','1','0','0','15';'AMK_TargetVelocity','16','16','LE','signed','Standard','0','1','0','0','65535';'AMK_TorqueLimitNegativ','48','16','LE','signed','Standard','0','1','0','0','65535';'AMK_TorqueLimitPositiv','32','16','LE','signed','Standard','0','1','0','0','65535';'AMK_bEnable','10','1','LE','unsigned','Standard','0','1','0','0','1';'AMK_bErrorReset','11','1','LE','unsigned','Standard','0','1','0','0','1';'AMK_bInverterOn','8','1','LE','unsigned','Standard','0','1','0','0','1';'AMK_bReserve','0','8','LE','unsigned','Standard','0','1','0','0','255';'CAN_bdcon','9','1','LE','unsigned','Standard','0','1','0','0','1'}
      settings: SourceProductBaseCode=ME,XP,VN  DataFormat=CANdb specified signals
  CAN Pack1 : canmsglib/CAN Pack  CANdbFile=D:\desktop\CANdbc\enable - youhou -.dbc  MsgList=(none)  MsgName=first_enable  MsgIDType=Standard (11-bit identifier)  MsgIdentifier=393  MsgLength=8  Remote=off  ApplyMinMax=off  BusOutput=off  SignalInfo={'AMK_Reserve','12','4','LE','signed','Standard','0','1','0','0','15';'AMK_TargetVelocity','16','16','LE','signed','Standard','0','1','0','0','65535';'AMK_TorqueLimitNegativ','48','16','LE','signed','Standard','0','1','0','0','65535';'AMK_TorqueLimitPositiv','32','16','LE','signed','Standard','0','1','0','0','65535';'AMK_bEnable','10','1','LE','unsigned','Standard','0','1','0','0','1';'AMK_bErrorReset','11','1','LE','unsigned','Standard','0','1','0','0','1';'AMK_bInverterOn','8','1','LE','unsigned','Standard','0','1','0','0','1';'AMK_bReserve','0','8','LE','unsigned','Standard','0','1','0','0','255';'CAN_bdcon','9','1','LE','unsigned','Standard','0','1','0','0','1'}
      settings: SourceProductBaseCode=ME,XP,VN  DataFormat=CANdb specified signals
  CANPackMessage : ec5744lib/RapidECU_U4B/04CANCommunication/CANPackMessage  datalength=8  sampletime=-1
      settings: SourceProductName=ECUCoder for MPC5744
  CANPackMessage1 : ec5744lib/RapidECU_U4B/04CANCommunication/CANPackMessage  datalength=8  sampletime=-1
      settings: SourceProductName=ECUCoder for MPC5744
  CANTransmit : ec5744lib/RapidECU_U4B/04CANCommunication/CANTransmit  canmodule=0  canbuffer=10  canmessageid=hex2dec('189')  canmessagetype=Standard(11-bit ID)  datalength=8  sampletime=-1
      settings: SourceProductName=ECUCoder for MPC5744
  Constant{,1..3,5,7..10,12,14,16..17} (13 alike) : Constant  Value=0  SampleTime=-1
  Constant{6,11,13,15} (4 alike) : Constant  SampleTime=-1
  Constant4 : Constant  Value=20000  SampleTime=-1
  Data Store Read1 : DataStoreRead  DataStoreName=Tzuohou
  Data Store Read2 : DataStoreRead  DataStoreName=lcu_enable_189
  Data Store Read3 : DataStoreRead  DataStoreName=lcu_enable_189_1
  Data Store Read5 : DataStoreRead  DataStoreName=yourenniuju
  Data Type Conversion : DataTypeConversion  OutDataTypeStr=uint8
  Data Type Conversion1 : DataTypeConversion  OutDataTypeStr=uint8
  MeaModule : ec5744lib/RapidECU_U4B/07Calibration/MeaModule  signal=T189
      settings: SourceProductName=ECUCoder for MPC5744
  MeaModule1 : ec5744lib/RapidECU_U4B/07Calibration/MeaModule  signal=Tthird
      settings: SourceProductName=ECUCoder for MPC5744
  Switch : Switch  Criteria=u2 > Threshold
  Switch1 : Switch  Criteria=u2 > Threshold
  Terminator : Terminator
  wires:
  Constant8/1 -> CAN Pack/8
  Constant5/1 -> CAN Pack/5
  Constant/1 -> CAN Pack/1
  CANPackMessage/1 -> Data Type Conversion/1
  Constant9/1 -> CAN Pack/9
  CAN Pack/1 -> CANPackMessage/1
  Constant7/1 -> CAN Pack/7
  Constant1/1 -> CAN Pack/2
  Constant16/1 -> CAN Pack/4
  Constant2/1 -> CAN Pack/3
  Constant6/1 -> CAN Pack/6
  CANTransmit/1 -> MeaModule/1
  MeaModule/1 -> Terminator/1
  Constant12/1 -> CAN Pack1/6
  Constant10/1 -> CAN Pack1/3
  Constant14/1 -> CAN Pack1/8
  Constant4/1 -> CAN Pack1/2
  Constant11/1 -> CAN Pack1/5
  Constant13/1 -> CAN Pack1/7
  CANPackMessage1/1 -> Data Type Conversion1/1
  CAN Pack1/1 -> CANPackMessage1/1
  Constant15/1 -> CAN Pack1/9
  Constant3/1 -> CAN Pack1/1
  Data Type Conversion1/1 -> Switch/1
  Data Type Conversion/1 -> Switch/3
  Switch/1 -> CANTransmit/1
  Data Store Read3/1 -> Switch/2
  MeaModule1/1 -> CAN Pack1/4
  Constant17/1 -> Switch1/3
  Data Store Read2/1 -> Switch1/2
  Switch1/1 -> MeaModule1/1
  Data Store Read1/1 -> Switch1/1

== system ultra/TX控制器/扭矩/TEST ==
  Data Store Read : DataStoreRead  Commented=on  DataStoreName=match_model
  MATLAB Function : MATLAB Function  Commented=on  TreatAsAtomicUnit=on
  Subsystem : Subsystem  Commented=on
  wires:
  Data Store Read/1 -> MATLAB Function/1(u)
  MATLAB Function/1(y) -> Subsystem/Enable

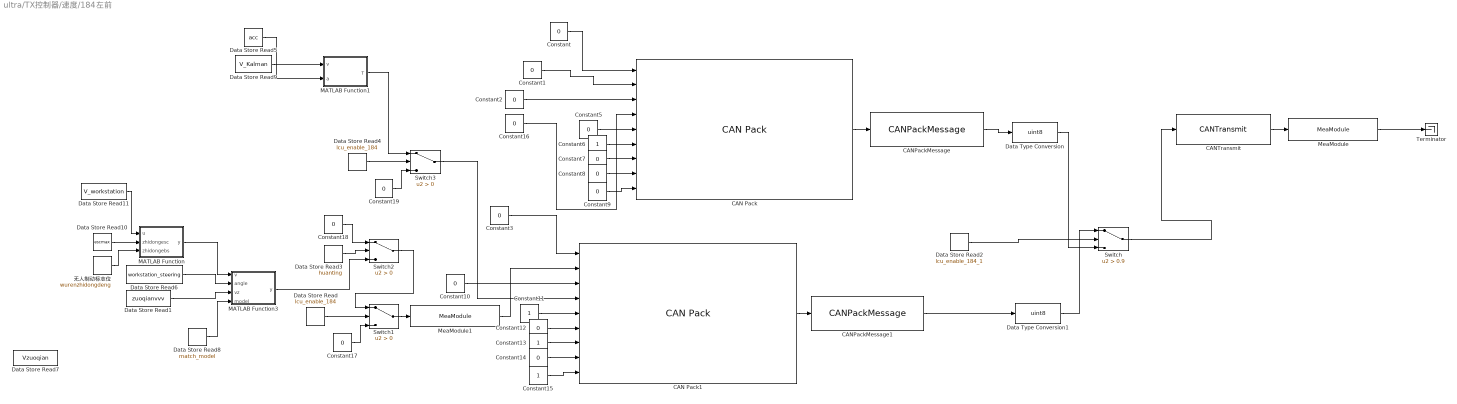
== system ultra/TX控制器/速度/184左前 ==
  CAN Pack : canmsglib/CAN Pack  CANdbFile=D:\desktop\CANdbc\enable.dbc  MsgList=(none)  MsgName=first_enable  MsgIDType=Standard (11-bit identifier)  MsgIdentifier=388  MsgLength=8  Remote=off  ApplyMinMax=off  BusOutput=off  SignalInfo={'AMK_Reserve','12','4','LE','signed','Standard','0','1','0','0','15';'AMK_TargetVelocity','16','16','LE','signed','Standard','0','1','0','0','65535';'AMK_TorqueLimitNegativ','48','16','LE','signed','Standard','0','1','0','0','65535';'AMK_TorqueLimitPositiv','32','16','LE','signed','Standard','0','1','0','0','65535';'AMK_bEnable','10','1','LE','unsigned','Standard','0','1','0','0','1';'AMK_bErrorReset','11','1','LE','unsigned','Standard','0','1','0','0','1';'AMK_bInverterOn','8','1','LE','unsigned','Standard','0','1','0','0','1';'AMK_bReserve','0','8','LE','unsigned','Standard','0','1','0','0','255';'CAN_bdcon','9','1','LE','unsigned','Standard','0','1','0','0','1'}
      settings: SourceProductBaseCode=ME,XP,VN  DataFormat=CANdb specified signals
  CAN Pack1 : canmsglib/CAN Pack  CANdbFile=D:\desktop\CANdbc\enable.dbc  MsgList=(none)  MsgName=first_enable  MsgIDType=Standard (11-bit identifier)  MsgIdentifier=388  MsgLength=8  Remote=off  ApplyMinMax=off  BusOutput=off  SignalInfo={'AMK_Reserve','12','4','LE','signed','Standard','0','1','0','0','15';'AMK_TargetVelocity','16','16','LE','signed','Standard','0','1','0','0','65535';'AMK_TorqueLimitNegativ','48','16','LE','signed','Standard','0','1','0','0','65535';'AMK_TorqueLimitPositiv','32','16','LE','signed','Standard','0','1','0','0','65535';'AMK_bEnable','10','1','LE','unsigned','Standard','0','1','0','0','1';'AMK_bErrorReset','11','1','LE','unsigned','Standard','0','1','0','0','1';'AMK_bInverterOn','8','1','LE','unsigned','Standard','0','1','0','0','1';'AMK_bReserve','0','8','LE','unsigned','Standard','0','1','0','0','255';'CAN_bdcon','9','1','LE','unsigned','Standard','0','1','0','0','1'}
      settings: SourceProductBaseCode=ME,XP,VN  DataFormat=CANdb specified signals
  CANPackMessage : ec5744lib/RapidECU_U4B/04CANCommunication/CANPackMessage  datalength=8  sampletime=-1
      settings: SourceProductName=ECUCoder for MPC5744
  CANPackMessage1 : ec5744lib/RapidECU_U4B/04CANCommunication/CANPackMessage  datalength=8  sampletime=-1
      settings: SourceProductName=ECUCoder for MPC5744
  CANTransmit : ec5744lib/RapidECU_U4B/04CANCommunication/CANTransmit  canmodule=0  canbuffer=8  canmessageid=hex2dec('184')  canmessagetype=Standard(11-bit ID)  datalength=8  sampletime=-1
      settings: SourceProductName=ECUCoder for MPC5744
  Constant{,1..3,5,7..10,12,14,16..17,19} (14 alike) : Constant  Value=0  SampleTime=-1
  Constant{6,11,13,15} (4 alike) : Constant  SampleTime=-1
  Constant18 : Constant  Value=0
  Data Store Read : DataStoreRead  DataStoreName=lcu_enable_184
  Data Store Read1 : DataStoreRead  DataStoreName=zuoqianvvv
  Data Store Read10 : DataStoreRead  DataStoreName=escmax
  Data Store Read11 : DataStoreRead  DataStoreName=V_workstation
  Data Store Read2 : DataStoreRead  DataStoreName=lcu_enable_184_1
  Data Store Read3 : DataStoreRead  DataStoreName=huanting
  Data Store Read4 : DataStoreRead  DataStoreName=lcu_enable_184
  Data Store Read5 : DataStoreRead  DataStoreName=acc
  Data Store Read6 : DataStoreRead  DataStoreName=workstation_steering
  Data Store Read7 : DataStoreRead  DataStoreName=Vzuoqian
  Data Store Read8 : DataStoreRead  DataStoreName=match_model
  Data Store Read9 : DataStoreRead  DataStoreName=V_Kalman
  Data Type Conversion : DataTypeConversion  OutDataTypeStr=uint8
  Data Type Conversion1 : DataTypeConversion  OutDataTypeStr=uint8
  MATLAB Function : MATLAB Function  TreatAsAtomicUnit=on
  MATLAB Function1 : MATLAB Function  TreatAsAtomicUnit=on
  MATLAB Function3 : MATLAB Function  TreatAsAtomicUnit=on
  MeaModule : ec5744lib/RapidECU_U4B/07Calibration/MeaModule  signal=V184
      settings: SourceProductName=ECUCoder for MPC5744
  MeaModule1 : ec5744lib/RapidECU_U4B/07Calibration/MeaModule  signal=Vfirst
      settings: SourceProductName=ECUCoder for MPC5744
  Switch : Switch  Criteria=u2 > Threshold  Threshold=0.9
  Switch1 : Switch  Criteria=u2 > Threshold
  Switch2 : Switch  Criteria=u2 > Threshold
  Switch3 : Switch  Criteria=u2 > Threshold
  Terminator : Terminator
  无人制动标志位 : DataStoreRead  DataStoreName=wurenzhidongdeng
  wires:
  Constant8/1 -> CAN Pack/8
  Constant5/1 -> CAN Pack/5
  Constant/1 -> CAN Pack/1
  Constant9/1 -> CAN Pack/9
  CAN Pack/1 -> CANPackMessage/1
  Constant7/1 -> CAN Pack/7
  Constant1/1 -> CAN Pack/2
  Constant16/1 -> CAN Pack/4
  Constant2/1 -> CAN Pack/3
  Constant6/1 -> CAN Pack/6
  CANTransmit/1 -> MeaModule/1
  MeaModule/1 -> Terminator/1
  Constant14/1 -> CAN Pack1/8
  Constant3/1 -> CAN Pack1/1
  Constant13/1 -> CAN Pack1/7
  CAN Pack1/1 -> CANPackMessage1/1
  Constant12/1 -> CAN Pack1/6
  CANPackMessage1/1 -> Data Type Conversion1/1
  Constant15/1 -> CAN Pack1/9
  Constant11/1 -> CAN Pack1/5
  Data Type Conversion1/1 -> Switch/1
  Constant10/1 -> CAN Pack1/3
  Switch/1 -> CANTransmit/1
  CANPackMessage/1 -> Data Type Conversion/1
  Data Type Conversion/1 -> Switch/3
  Switch1/1 -> MeaModule1/1
  Data Store Read/1 -> Switch1/2
  Constant17/1 -> Switch1/3
  Data Store Read2/1 -> Switch/2
  Data Store Read3/1 -> Switch2/2
  Constant18/1 -> Switch2/1
  Switch2/1 -> Switch1/1
  MeaModule1/1 -> CAN Pack1/2
  Data Store Read4/1 -> Switch3/2
  Constant19/1 -> Switch3/3
  Switch3/1 -> CAN Pack1/4
  Data Store Read5/1 -> MATLAB Function1/2(a)
  MATLAB Function1/1(T) -> Switch3/1
  MATLAB Function/1(y) -> MATLAB Function3/1(v)
  MATLAB Function3/1(y) -> Switch2/3
  Data Store Read6/1 -> MATLAB Function3/2(angle)
  Data Store Read8/1 -> MATLAB Function3/4(model)
  Data Store Read9/1 -> MATLAB Function1/1(v)
  Data Store Read10/1 -> MATLAB Function/2(zhidongesc)
  无人制动标志位/1 -> MATLAB Function/3(zhidongebs)
  Data Store Read11/1 -> MATLAB Function/1(u)
  Data Store Read1/1 -> MATLAB Function3/3(vz)
